simulink library "models2"  (Simulink 6.0)
values from neighbouring files (symbols this model uses):
  width = abs(diff(LTRB(1:2:3)))    [LTRB2Centre.m]
undefined symbols (not defined in the file or in its folder): beta, C, center, coeffs, delG, exponent, i, initialYValues, interact, invcodeData, invDG, knots, m, maxDelay, n, nhi, nk, nlo, numInputSignals, numterms, orderM, paramIndex, poly_order, polycoeff, polyTerms, reorderM, S, s0, s1, sampleTime, target, WendlandNumTerms, Xvalues
libraries: models2 x45, simulink x17
(part 1 of 2)
settings Model: Creator=ralcock  LastModifiedBy=ralcock  ExtModeAutoUpdateStatusClock=off

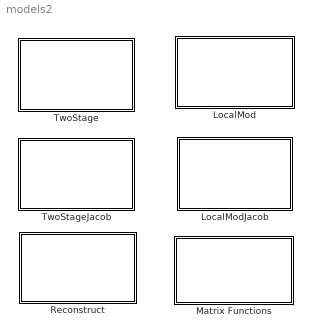
== system models2 ==
  LocalMod : Subsystem
      mask Display: disp('Local Models')
  LocalModJacob : Subsystem
      mask Display: disp('Local Model Jacobians')
  Matrix Functions : Subsystem
      mask Display: disp('Matrix Functions')
  Reconstruct : Subsystem
      mask Display: disp('LocalMod Reconstruct')
  TwoStage : Subsystem
      mask Display: disp('Two Stage models')
  TwoStageJacob : Subsystem
      mask Display: disp('Two Stage Jacobians')

== system models2/LocalMod ==
  expGrowthEval : Subsystem
  gompEval : Subsystem
  localSurfaceCubicEval : Subsystem
  localSurfaceSplineEval : Subsystem  AncestorBlock=models2/TwoStage/xreg3xSplineEval
  localbsplineEval : Subsystem
  logistic4Eval : Subsystem
  logisticEval : Subsystem
  mmfEval : Subsystem
  polynomEval : Subsystem
  polysplineEval : Subsystem
  quadsplineEval : Subsystem
  richardEval : Subsystem
  truncpsEval : Subsystem
  userLocalEval : Subsystem
  weibulEval : Subsystem

== system models2/LocalModJacob ==
  PolynomJacob : Subsystem
  expgrowthJacob : Subsystem
  gompJacob : Subsystem
  localSurfaceCubicJacob : Subsystem  AncestorBlock=models2/TwoStageJacob/xregcubicJacob
  localSurfaceSplineJacob : Subsystem  AncestorBlock=models2/TwoStageJacob/xreg3xsplineJacob
  logistic4Jacob : Subsystem
  logisticJacob : Subsystem
  mmfJacob : Subsystem
  polysplineJacob : Subsystem
  richardJacob : Subsystem
  userLocalJacob : Subsystem
  weibulJacob : Subsystem

== system models2/Matrix Functions ==
  mvMultiplyMatrixSFn : S-Function  FunctionName=mvMultiplyMatrixSFnV1  Parameters=s0,s1
      mask Display: disp('X*Y')
  mvTransposeMatrixSFn : S-Function  FunctionName=mvTransposeMatrixSFnV1  Parameters=s0
      mask Display: disp('X''')

== system models2/Reconstruct ==
  gompRecon : Subsystem
  linearRecon : Subsystem
  localBSplineRecon : Subsystem
  localtruncpsRecon : Subsystem
  log4Recon : Subsystem
  logRecon : Subsystem
  mmfRecon : Subsystem
  richReconDelta : Subsystem
  richReconKappa : Subsystem
  userLocalRecon : Subsystem
  weibRecon : Subsystem

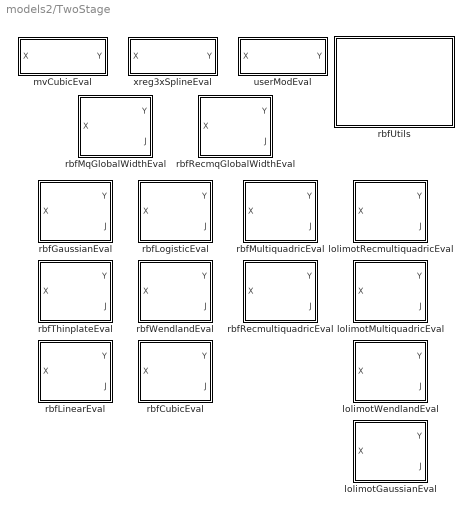
== system models2/TwoStage ==
  lolimotGaussianEval : Subsystem  mask{P=polycoeff, S=width, C=center}
      mask prompts: P "Polynomial coeficients"; S "Widths"; C "Centers"
  lolimotMultiquadricEval : Subsystem  mask{P=polycoeff, S=width, C=center}
      mask prompts: P "Polynomial coeficients"; S "Widths"; C "Centers"
  lolimotRecmultiquadricEval : Subsystem  mask{P=polycoeff, S=width, C=center}
      mask prompts: P "Polynomial coeficients"; S "Widths"; C "Centers"
  lolimotWendlandEval : Subsystem  mask{WendlandNumTerms=WendlandNumTerms, E=exponent, WP=polyTerms, P=polycoeff, S=width, C=center}
      mask prompts: WendlandNumTerms "Number of Polynomial Terms"; E "Exponent"; WP "Polynomial Terms"; P "Polynomial coeficients"; S "Widths"; C "Centers"
  mvCubicEval : Subsystem  AncestorBlock=models2/TwoStage/userModEval
  rbfCubicEval : Subsystem  AncestorBlock=models2/TwoStage/rbfLinearEval  mask{B=beta, S=width, C=center}
      mask prompts: B "Betas"; S "Widths"; C "Centers"
  rbfGaussianEval : Subsystem  mask{B=beta, S=width, C=center}
      mask prompts: B "Betas"; S "Widths"; C "Centers"
  rbfLinearEval : Subsystem  AncestorBlock=models2/TwoStage/rbfThinplateEval  mask{B=beta, S=width, C=center}
      mask prompts: B "Betas"; S "Widths"; C "Centers"
  rbfLogisticEval : Subsystem  mask{B=beta, S=width, C=center}
      mask prompts: B "Betas"; S "Widths"; C "Centers"
  rbfMqGlobalWidthEval : Subsystem  AncestorBlock=models2/TwoStage/rbfMultiquadricEval  mask{B=beta, S=width, C=center}
      mask prompts: B "Betas"; S "Widths"; C "Centers"
  rbfMultiquadricEval : Subsystem  mask{B=beta, S=width, C=center}
      mask prompts: B "Betas"; S "Widths"; C "Centers"
  rbfRecmqGlobalWidthEval : Subsystem  AncestorBlock=models2/TwoStage/rbfRecmultiquadricEval  mask{B=beta, S=width, C=center}
      mask prompts: B "Betas"; S "Widths"; C "Centers"
  rbfRecmultiquadricEval : Subsystem  mask{B=beta, S=width, C=center}
      mask prompts: B "Betas"; S "Widths"; C "Centers"
  rbfThinplateEval : Subsystem  mask{B=beta, S=width, C=center}
      mask prompts: B "Betas"; S "Widths"; C "Centers"
  rbfUtils : Subsystem
      mask Display: disp('RBF Utility blocks')
  rbfWendlandEval : Subsystem  mask{NumTerms=WendlandNumTerms, E=exponent, P=polyTerms, B=beta, S=width, C=center}
      mask prompts: NumTerms "Number of Poylnomial Terms"; E "Exponent"; P "Polynomial Terms"; B "Betas"; S "Widths"; C "Centers"
  userModEval : Subsystem
  xreg3xSplineEval : Subsystem

== system models2/TwoStageJacob ==
  lollimotJacob : Subsystem
  mvcubicJacob : Subsystem
      mask Display: disp('mvCubicJacob')
  rbfJacob : Subsystem
  userModJacob : Subsystem
  xreg3xsplineJacob : Subsystem
      mask Display: disp('xreg3xSplineJacob')
  xregJacob : models2/TwoStageJacob/rbfJacob
  xregcubicJacob : Subsystem  AncestorBlock=models2/TwoStageJacob/mvcubicJacob
      mask Display: disp('mvCubicJacob')
  xreglinear_x2fx : Subsystem
  xregusermodJacob : models2/TwoStageJacob/userModJacob

== system models2/LocalMod/expGrowthEval ==
  P : Inport
  X : Inport  Port=2
  Demux : Demux  Outputs=3
  Gain : Gain  Gain=-1  SaturateOnIntegerOverflow=on
  Math Function : Math  SaturateOnIntegerOverflow=on
  Product : Product  SaturateOnIntegerOverflow=on  InputSameDT=on
  Product1 : Product  SaturateOnIntegerOverflow=on  InputSameDT=on
  Sum : Sum  Inputs=|+-  SaturateOnIntegerOverflow=on  InputSameDT=on
  Sum1 : Sum  Inputs=+-|  SaturateOnIntegerOverflow=on  InputSameDT=on
  Y : Outport
  wires:
  P/1 -> Demux/1
  Demux/2 -> Sum/2  "b"
  Demux/1 -> Sum/1, Sum1/1  "a"
  X/1 -> Product1/2
  Demux/3 -> Gain/1  "k"
  Gain/1 -> Product1/1
  Product1/1 -> Math Function/1
  Math Function/1 -> Product/2
  Sum/1 -> Product/1
  Product/1 -> Sum1/2
  Sum1/1 -> Y/1

== system models2/LocalMod/gompEval ==
  note: a
  note: g
  note: k
  P : Inport
  X : Inport  Port=2
  Demux : Demux  Outputs=3
  Gain : Gain  Gain=-1  SaturateOnIntegerOverflow=on
  Gain1 : Gain  Gain=-1  SaturateOnIntegerOverflow=on
  Math Function : Math  SaturateOnIntegerOverflow=on
  Math Function1 : Math  SaturateOnIntegerOverflow=on
  Product : Product  SaturateOnIntegerOverflow=on  InputSameDT=on
  Product1 : Product  SaturateOnIntegerOverflow=on  InputSameDT=on
  Sum : Sum  Inputs=|-+  SaturateOnIntegerOverflow=on  InputSameDT=on
  Y : Outport
  wires:
  P/1 -> Demux/1
  Demux/2 -> Sum/1
  Demux/3 -> Gain/1
  X/1 -> Sum/2
  Sum/1 -> Product/1
  Gain/1 -> Product/2
  Product/1 -> Math Function/1
  Math Function/1 -> Gain1/1
  Gain1/1 -> Math Function1/1
  Math Function1/1 -> Product1/2
  Demux/1 -> Product1/1
  Product1/1 -> Y/1

== system models2/LocalMod/localSurfaceCubicEval ==
  P : Inport
  X : Inport  Port=2
  Assignment : Assignment  Elements=termsin
  Constant1 : Constant  Value=zeros(1, numterms)
  S-Function : models2/TwoStage/mvCubicEval/S-Function
  Y : Outport
  wires:
  S-Function/1 -> Y/1
  X/1 -> S-Function/2
  P/1 -> Assignment/2
  Assignment/1 -> S-Function/1
  Constant1/1 -> Assignment/1

== system models2/LocalMod/localSurfaceSplineEval ==
  P1 : Inport
  X : Inport  Port=2
  Assignment : Assignment  Elements=termsin
  Constant1 : Constant  Value=zeros(1, numterms)
  S-Function : models2/TwoStage/xreg3xSplineEval/S-Function
  Y : Outport
  wires:
  X/1 -> S-Function/2
  S-Function/1 -> Y/1
  P1/1 -> Assignment/2
  Assignment/1 -> S-Function/1
  Constant1/1 -> Assignment/1

== system models2/LocalMod/localbsplineEval ==
  P : Inport
  X : Inport  Port=2
  S-Function : S-Function  FunctionName=LocalBSplineEvalSFnV1  Parameters="orderm, reorderm,  knots, poly_order, interact, limits"  SFunctionModules=xregsimulinkutils
  Y : Outport
  wires:
  X/1 -> S-Function/2
  S-Function/1 -> Y/1
  P/1 -> S-Function/1

== system models2/LocalMod/logistic4Eval ==
  note: -k * (log(x) - g
  P : Inport
  X : Inport  Port=2
  Constant : Constant
  Demux : Demux
  Gain : Gain  Gain=-1  SaturateOnIntegerOverflow=on
  Math Function : Math  Operator=log  SaturateOnIntegerOverflow=on
  Math Function1 : Math  SaturateOnIntegerOverflow=on
  Product : Product  Inputs=*/  SaturateOnIntegerOverflow=on  InputSameDT=on
  Product1 : Product  SaturateOnIntegerOverflow=on  InputSameDT=on
  Sum : Sum  Inputs=-+|  SaturateOnIntegerOverflow=on  InputSameDT=on
  Sum1 : Sum  Inputs=+-|  SaturateOnIntegerOverflow=on  InputSameDT=on
  Sum2 : Sum  Inputs=|-+  SaturateOnIntegerOverflow=on  InputSameDT=on
  Sum3 : Sum  Inputs=|++  SaturateOnIntegerOverflow=on  InputSameDT=on
  Y : Outport
  wires:
  Demux/2 -> Sum1/1, Sum/2  "b"
  Sum1/1 -> Y/1
  Product/1 -> Sum1/2
  Sum/1 -> Product/1
  Demux/1 -> Sum/1  "a"
  Sum2/1 -> Product1/2
  Math Function/1 -> Sum2/2
  Demux/4 -> Sum2/1  "g"
  Gain/1 -> Product1/1
  Sum3/1 -> Product/2
  Constant/1 -> Sum3/2
  Math Function1/1 -> Sum3/1
  Product1/1 -> Math Function1/1
  Demux/3 -> Gain/1  "k"
  X/1 -> Math Function/1
  P/1 -> Demux/1

== system models2/LocalMod/logisticEval ==
  P : Inport
  X : Inport  Orientation=up  Port=2
  Constant : Constant  Orientation=up
  Demux : Demux  Outputs=3
  Gain : Gain  Gain=-1  SaturateOnIntegerOverflow=on
  Math Function : Math  SaturateOnIntegerOverflow=on
  Product : Product  SaturateOnIntegerOverflow=on  InputSameDT=on
  Product1 : Product  Inputs=*/  SaturateOnIntegerOverflow=on  InputSameDT=on
  Sum : Sum  Inputs=|-+  SaturateOnIntegerOverflow=on  InputSameDT=on
  Sum1 : Sum  Inputs=|++  SaturateOnIntegerOverflow=on  InputSameDT=on
  Y : Outport
  wires:
  P/1 -> Demux/1
  Demux/2 -> Sum/1  "g"
  Demux/3 -> Gain/1  "k"
  X/1 -> Sum/2
  Gain/1 -> Product/2
  Sum/1 -> Product/1
  Product/1 -> Math Function/1
  Math Function/1 -> Sum1/1
  Constant/1 -> Sum1/2
  Sum1/1 -> Product1/2
  Demux/1 -> Product1/1  "a"
  Product1/1 -> Y/1

== system models2/LocalMod/mmfEval ==
  P : Inport
  X : Inport  Orientation=up  Port=2
  Constant : Constant  Orientation=down
  Constant1 : Constant  Orientation=down  Value=NaN
  Constant2 : Constant  Value=0
  Data Type Conversion : DataTypeConversion  OutDataTypeMode=boolean  SaturateOnIntegerOverflow=on  RndMeth=Zero
  Demux : Demux
  Logical Operator : Logic  Operator=OR
  Product : Product  SaturateOnIntegerOverflow=on  InputSameDT=on
  Product1 : Product  Inputs=*/  SaturateOnIntegerOverflow=on  InputSameDT=on
  Relational Operator : RelationalOperator  Operator=<  InputSameDT=on
  SubSystem : Subsystem
  Sum : Sum  Inputs=|+-  SaturateOnIntegerOverflow=on  InputSameDT=on
  Sum2 : Sum  Inputs=+-|  SaturateOnIntegerOverflow=on  InputSameDT=on
  Sum3 : Sum  Inputs=++|  SaturateOnIntegerOverflow=on  InputSameDT=on
  Switch : Switch  Criteria=u2 ~= 0  SaturateOnIntegerOverflow=on  InputSameDT=on
  isComplex : Probe  ProbeWidth=off  ProbeSampleTime=off
  Y : Outport
  wires:
  P/1 -> Demux/1
  Demux/2 -> Sum/2  "b"
  Demux/3 -> Product/1  "k"
  X/1 -> Product/2, Relational Operator/1
  Product/1 -> SubSystem/1(U)
  Sum/1 -> Product1/1
  Product1/1 -> Sum2/2
  Demux/1 -> Sum2/1, Sum/1  "a"
  Demux/4 -> SubSystem/2(V)  "d"
  Switch/1 -> Y/1
  Sum2/1 -> Switch/3, isComplex/1
  Constant1/1 -> Switch/1
  SubSystem/1(U^V) -> Sum3/2
  Constant/1 -> Sum3/1
  Sum3/1 -> Product1/2
  Constant2/1 -> Relational Operator/2
  isComplex/1 -> Data Type Conversion/1
  Logical Operator/1 -> Switch/2
  Relational Operator/1 -> Logical Operator/2
  Data Type Conversion/1 -> Logical Operator/1

== system models2/LocalMod/polynomEval ==
  P : Inport
  X : Inport  Port=2
  polynomEval : S-Function  FunctionName=PolynomEvalSFnV1
  Y : Outport
  wires:
  P/1 -> polynomEval/1
  polynomEval/1 -> Y/1
  X/1 -> polynomEval/2

== system models2/LocalMod/polysplineEval ==
  P : Inport
  X : Inport  Port=2
  datum : Inport  Port=3
  Demux : Demux  Outputs=[1 1 nhi nlo]
  Linear term : Constant  Orientation=down  Value=0
  Mux : Mux  Inputs=3
  Mux1 : Mux  Inputs=3
  Selector : Selector  Elements=[nhi:-1:1]  InputPortWidth=nhi
  Selector1 : Selector  Elements=[nlo:-1:1]  InputPortWidth=nlo
  Sum : Sum  Inputs=-+|  SaturateOnIntegerOverflow=on  InputSameDT=on
  Sum4 : Sum  Inputs=-+|  SaturateOnIntegerOverflow=on  InputSameDT=on
  Switch : Switch  Threshold=eps  InputSameDT=on
  polynomEval1 : S-Function  FunctionName=PolynomEvalSFnV1
  polynomEval2 : S-Function  FunctionName=PolynomEvalSFnV1
  local : Outport
  wires:
  P/1 -> Demux/1
  Demux/3 -> Selector/1  "Phigh"
  Demux/4 -> Selector1/1  "Plow"
  datum/1 -> Sum4/1
  Demux/1 -> Sum4/2  "knot"
  X/1 -> Sum/2
  Sum4/1 -> Sum/1
  Selector/1 -> Mux/1
  Mux/1 -> polynomEval1/1
  Sum/1 -> polynomEval2/2, polynomEval1/2, Switch/2  "X-k"
  Selector1/1 -> Mux1/1
  Mux1/1 -> polynomEval2/1
  Linear term/1 -> Mux/2, Mux1/2
  Demux/2 -> Mux/3, Mux1/3  "P0"
  Switch/1 -> local/1
  polynomEval1/1 -> Switch/1
  polynomEval2/1 -> Switch/3

== system models2/LocalMod/quadsplineEval ==
  note: (X-knot)
  note: (X-knot).^2
  note: quadlow
  note: X
  note: quadhigh
  note: (X-knot).^2
  note: X
  P : Inport
  X : Inport  Port=2
  datum : Inport  Port=3
  Demux : Demux
  Math Function : Math  Operator=square  SaturateOnIntegerOverflow=on
  Math Function1 : Math  Operator=square  SaturateOnIntegerOverflow=on
  Product : Product  SaturateOnIntegerOverflow=on  InputSameDT=on
  Product1 : Product  SaturateOnIntegerOverflow=on  InputSameDT=on
  Sum : Sum  Inputs=|+-  SaturateOnIntegerOverflow=on  InputSameDT=on
  Sum1 : Sum  Inputs=|++  SaturateOnIntegerOverflow=on  InputSameDT=on
  Sum2 : Sum  Inputs=-+|  SaturateOnIntegerOverflow=on  InputSameDT=on
  Sum3 : Sum  Inputs=++|  SaturateOnIntegerOverflow=on  InputSameDT=on
  Sum4 : Sum  Inputs=-+|  SaturateOnIntegerOverflow=on  InputSameDT=on
  Switch : Switch  Threshold=eps  InputSameDT=on
  local : Outport
  wires:
  Switch/1 -> local/1
  Sum/1 -> Switch/2, Math Function/1
  Product1/1 -> Sum3/2
  Demux/4 -> Product1/1  "Plow"
  Math Function1/1 -> Product1/2
  Sum2/1 -> Math Function1/1
  X/1 -> Sum2/2, Sum/1
  Product/1 -> Sum1/1
  Demux/3 -> Product/2  "Phigh"
  P/1 -> Demux/1
  Math Function/1 -> Product/1
  Demux/2 -> Sum3/1, Sum1/2  "P0"
  Sum3/1 -> Switch/3
  Sum1/1 -> Switch/1
  Demux/1 -> Sum4/2  "knot"
  datum/1 -> Sum4/1
  Sum4/1 -> Sum/2, Sum2/1

== system models2/LocalMod/richardEval ==
  note: The Tolerance block triggers when
      | d is within 3e-6 of 1. See notes from
      |  TM for a definition of the limit at d =1
  P : Inport
  X : Inport  Port=2
  Complex to Real-Imag : ComplexToRealImag  Output=Real
  Complex to Real-Imag1 : ComplexToRealImag  Output=Imag
  Constant1 : Constant  Orientation=down  Value=NaN + i
  Data Type Conversion : DataTypeConversion  OutDataTypeMode=boolean  SaturateOnIntegerOverflow=on  RndMeth=Zero
  Demux1 : Demux
  Logical Operator : Logic  Operator=NOT
  Richards : Subsystem  TreatAsAtomicUnit=on
  Richards  at d == 1 : Subsystem  TreatAsAtomicUnit=on
  SubSystem : models2/LocalModJacob/richardJacob/SubSystem  V=1  T=3e-6
  Switch : Switch  Threshold=0.5  InputSameDT=on
  Switch1 : Switch  Criteria=u2 ~= 0  SaturateOnIntegerOverflow=on  InputSameDT=on
  Terminator1 : Terminator
  Terminator2 : Terminator
  Terminator3 : Terminator
  Y : Outport
  wires:
  Demux1/4 -> SubSystem/1  "d"
  P/1 -> Richards/1(P), Richards  at d == 1/1(P), Demux1/1
  X/1 -> Richards/2(X), Richards  at d == 1/2(X)
  Richards  at d == 1/1(Y) -> Switch/3
  Richards/1(Y) -> Switch/1
  Demux1/1 -> Terminator2/1  "a"
  Demux1/2 -> Terminator1/1  "g"
  Demux1/3 -> Terminator3/1  "k"
  SubSystem/1 -> Logical Operator/1, Richards  at d == 1/Enable
  Logical Operator/1 -> Switch/2, Richards/Enable
  Switch1/1 -> Complex to Real-Imag/1
  Constant1/1 -> Switch1/1
  Complex to Real-Imag1/1 -> Data Type Conversion/1
  Switch/1 -> Switch1/3, Complex to Real-Imag1/1
  Data Type Conversion/1 -> Switch1/2
  Complex to Real-Imag/1 -> Y/1

== system models2/LocalMod/truncpsEval ==
  P : Inport
  X : Inport  Port=2
  Constant1 : Constant  Value=m
  Constant2 : Constant  Value=0
  Demux : Demux  Outputs=[nk n-2*nk nk]
  Dot Product : simulink/Math Operations/Dot Product  OutDataType=sfix(16)  OutScaling=2^-10  DoSatur=off
  Math Function : Math  Operator=pow  SaturateOnIntegerOverflow=on
  Sum : Sum  Inputs=|+-  SaturateOnIntegerOverflow=on  InputSameDT=on
  Sum2 : Sum  Inputs=++|  SaturateOnIntegerOverflow=on  InputSameDT=on
  Switch : Switch  InputSameDT=on
  polyval : S-Function  FunctionName=PolynomEvalSFnV1
  y : Outport
  wires:
  Demux/2 -> polyval/1  "b_poly"
  Sum2/1 -> y/1
  polyval/1 -> Sum2/1
  Constant1/1 -> Math Function/2
  Switch/1 -> Math Function/1
  Dot Product/1 -> Sum2/2
  Math Function/1 -> Dot Product/1
  Demux/3 -> Dot Product/2  "bspline"
  Constant2/1 -> Switch/3
  X/1 -> Sum/1, polyval/2
  Sum/1 -> Switch/2, Switch/1
  P/1 -> Demux/1
  Demux/1 -> Sum/2  "knots"

== system models2/LocalMod/userLocalEval ==
  P : Inport
  X : Inport  Port=2
  Y : Outport

== system models2/LocalMod/weibulEval ==
  P : Inport
  X : Inport  Orientation=up  Port=2
  Constant1 : Constant  Orientation=down  Value=NaN
  Constant2 : Constant  Value=0
  Data Type Conversion : DataTypeConversion  OutDataTypeMode=boolean  SaturateOnIntegerOverflow=on  RndMeth=Zero
  Demux : Demux
  Logical Operator : Logic  Operator=OR
  Product : Product  SaturateOnIntegerOverflow=on  InputSameDT=on
  Product1 : Product  SaturateOnIntegerOverflow=on  InputSameDT=on
  Relational Operator : RelationalOperator  Operator=<  InputSameDT=on
  SubSystem : Subsystem
  Sum : Sum  Inputs=+-|  SaturateOnIntegerOverflow=on  InputSameDT=on
  Sum1 : Sum  Inputs=+-|  SaturateOnIntegerOverflow=on  InputSameDT=on
  Switch : Switch  Criteria=u2 ~= 0  SaturateOnIntegerOverflow=on  InputSameDT=on
  isComplex : Probe  ProbeWidth=off  ProbeSampleTime=off
  Y : Outport
  wires:
  Product1/1 -> Sum1/2
  Sum/1 -> Product1/1
  SubSystem/1(e^-(U^V)) -> Product1/2  "-(k*x) ^ d"
  Product/1 -> SubSystem/1(U)
  Demux/1 -> Sum1/1, Sum/1  "a"
  Demux/2 -> Sum/2  "b"
  Demux/4 -> SubSystem/2(V)  "d"
  X/1 -> Product/2, Relational Operator/1
  Demux/3 -> Product/1  "k"
  P/1 -> Demux/1
  Constant1/1 -> Switch/1
  isComplex/1 -> Data Type Conversion/1
  Logical Operator/1 -> Switch/2
  Constant2/1 -> Relational Operator/2
  Sum1/1 -> Switch/3, isComplex/1
  Switch/1 -> Y/1
  Relational Operator/1 -> Logical Operator/2
  Data Type Conversion/1 -> Logical Operator/1

== system models2/LocalModJacob/PolynomJacob ==
  P : Inport
  X : Inport  Port=2
  PolynomJacob : S-Function  FunctionName=PolynomJacobSFnV1
  J : Outport
  wires:
  PolynomJacob/1 -> J/1
  X/1 -> PolynomJacob/2
  P/1 -> PolynomJacob/1

== system models2/LocalModJacob/expgrowthJacob ==
  P : Inport
  X : Inport  Port=2
  Constant : Constant
  Demux : Demux  Outputs=3
  Gain : Gain  Gain=-1  SaturateOnIntegerOverflow=on
  Gain3 : Gain  Gain=-1  SaturateOnIntegerOverflow=on
  Math Function : Math  SaturateOnIntegerOverflow=on
  Mux : Mux  Inputs=3
  Product1 : Product  SaturateOnIntegerOverflow=on  InputSameDT=on
  Product2 : Product  Inputs=3  SaturateOnIntegerOverflow=on  InputSameDT=on
  Sum : Sum  Inputs=|+-  SaturateOnIntegerOverflow=on  InputSameDT=on
  Sum1 : Sum  Inputs=|+-  SaturateOnIntegerOverflow=on  InputSameDT=on
  J : Outport
  wires:
  Demux/3 -> Gain/1  "k"
  Demux/1 -> Sum/1  "a"
  Demux/2 -> Sum/2  "b"
  Sum1/1 -> Mux/1  "Ja"
  Sum/1 -> Product2/3
  X/1 -> Product1/2, Product2/2
  Product2/1 -> Mux/3  "Jk"
  Gain/1 -> Product1/1
  Product1/1 -> Math Function/1
  Math Function/1 -> Sum1/2, Mux/2, Product2/1  "Jb"
  Gain3/1 -> J/1
  Mux/1 -> Gain3/1
  P/1 -> Demux/1
  Constant/1 -> Sum1/1

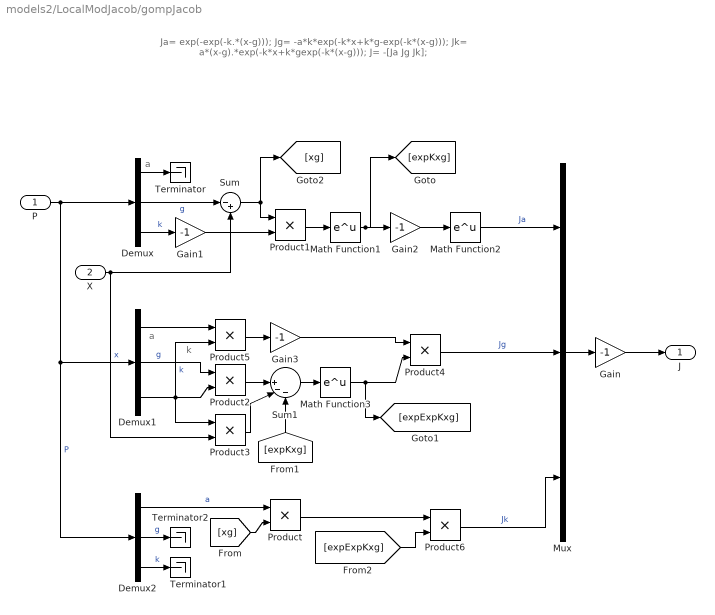
== system models2/LocalModJacob/gompJacob ==
  note: Ja= exp(-exp(-k.*(x-g)));
      | Jg= -a*k*exp(-k*x+k*g-exp(-k*(x-g)));
      | Jk= a*(x-g).*exp(-k*x+k*gexp(-k*(x-g)));
      |
      | J= -[Ja Jg Jk];
  note: a
  note: a
  note: k
  P : Inport
  X : Inport  Port=2
  Demux : Demux  Outputs=3
  Demux1 : Demux  Outputs=3
  Demux2 : Demux  Outputs=3
  Gain{,1..3} (4 alike) : Gain  Gain=-1  SaturateOnIntegerOverflow=on
  Math Function1 : Math  SaturateOnIntegerOverflow=on
  Math Function2 : Math  SaturateOnIntegerOverflow=on
  Math Function3 : Math  SaturateOnIntegerOverflow=on
  Mux : Mux  Inputs=3
  Product{,1..6} (7 alike) : Product  SaturateOnIntegerOverflow=on  InputSameDT=on
  Sum : Sum  Inputs=|-+  SaturateOnIntegerOverflow=on  InputSameDT=on
  Sum1 : Sum  Inputs=||+--  SaturateOnIntegerOverflow=on  InputSameDT=on
  Terminator : Terminator
  Terminator1 : Terminator
  Terminator2 : Terminator
  J : Outport
  wires:
  Gain/1 -> J/1
  Demux/1 -> Terminator/1
  Demux/2 -> Sum/1  "g"
  Product1/1 -> Math Function1/1
  Demux/3 -> Gain1/1  "k"
  Gain1/1 -> Product1/2
  Gain2/1 -> Math Function2/1
  Math Function1/1 -> Gain2/1, [expKxg]
  P/1 -> Demux/1, Demux1/1, Demux2/1  "P"
  X/1 -> Sum/2, Product3/2  "x"
  Sum/1 -> Product1/1, [xg]
  Demux2/3 -> Terminator1/1  "k"
  Demux2/2 -> Terminator2/1  "g"
  Demux2/1 -> Product/1  "a"
  [xg] -> Product/2
  Product/1 -> Product6/1
  [expExpKxg] -> Product6/2
  Product6/1 -> Mux/3  "Jk"
  Math Function2/1 -> Mux/1  "Ja"
  Mux/1 -> Gain/1
  Demux1/2 -> Product2/1  "g"
  Product2/1 -> Sum1/1
  [expKxg] -> Sum1/3
  Demux1/3 -> Product3/1, Product2/2, Product5/2  "k"
  Product3/1 -> Sum1/2
  Sum1/1 -> Math Function3/1
  Math Function3/1 -> [expExpKxg], Product4/2
  Demux1/1 -> Product5/1
  Product5/1 -> Gain3/1
  Gain3/1 -> Product4/1
  Product4/1 -> Mux/2  "Jg"

== system models2/LocalModJacob/localSurfaceCubicJacob ==
  P1 : Inport
  X : Inport  Port=2
  Assignment : Assignment  Elements=termsin
  Constant1 : Constant  Value=zeros(1, numterms)
  S-Function : models2/TwoStageJacob/xregcubicJacob/S-Function
  Selector1 : Selector  Elements=termsout  InputPortWidth=numterms
  J : Outport
  wires:
  S-Function/1 -> Selector1/1
  X/1 -> S-Function/2
  Selector1/1 -> J/1
  P1/1 -> Assignment/2
  Assignment/1 -> S-Function/1
  Constant1/1 -> Assignment/1

== system models2/LocalModJacob/localSurfaceSplineJacob ==
  P : Inport
  X : Inport  Port=2
  Assignment : Assignment  Elements=termsin
  Constant1 : Constant  Value=zeros(1, numterms)
  S-Function : models2/TwoStageJacob/xreg3xsplineJacob/S-Function
  Selector1 : Selector  Elements=termsout  InputPortWidth=numterms
  J : Outport
  wires:
  S-Function/1 -> Selector1/1
  X/1 -> S-Function/2
  Selector1/1 -> J/1
  P/1 -> Assignment/2
  Assignment/1 -> S-Function/1
  Constant1/1 -> Assignment/1

== system models2/LocalModJacob/logistic4Jacob ==
  P : Inport
  X : Inport  Port=2
  Constant : Constant  Orientation=down
  Demux : Demux
  Demux1 : Demux  Outputs=3
  Gain : Gain  Gain=-1  SaturateOnIntegerOverflow=on
  Gain2 : Gain  Gain=-1  SaturateOnIntegerOverflow=on
  Math Function : Math  Operator=log  SaturateOnIntegerOverflow=on
  Mux : Mux  Inputs=3
  Mux1 : Mux
  Sum : Sum  Inputs=-+|  SaturateOnIntegerOverflow=on  InputSameDT=on
  Sum1 : Sum  Inputs=-+|  SaturateOnIntegerOverflow=on  InputSameDT=on
  logisticJacob : Subsystem
  J : Outport
  wires:
  P/1 -> Demux/1
  Demux/1 -> Sum/1  "a"
  Demux/2 -> Sum/2  "b"
  Sum/1 -> Mux/1  "a'"
  Mux/1 -> logisticJacob/1(P)
  Demux/3 -> Mux/3  "k"
  Demux/4 -> Mux/2  "g"
  X/1 -> Math Function/1
  Math Function/1 -> logisticJacob/2(X)
  Demux1/1 -> Sum1/2, Gain/1  "Ja"
  Constant/1 -> Sum1/1
  Sum1/1 -> Mux1/2  "Jb"
  Mux1/1 -> J/1
  Demux1/2 -> Mux1/4  "Jg"
  Demux1/3 -> Mux1/3  "Jk"
  Gain/1 -> Mux1/1  "Ja"
  logisticJacob/1(J) -> Gain2/1
  Gain2/1 -> Demux1/1  "Ja"

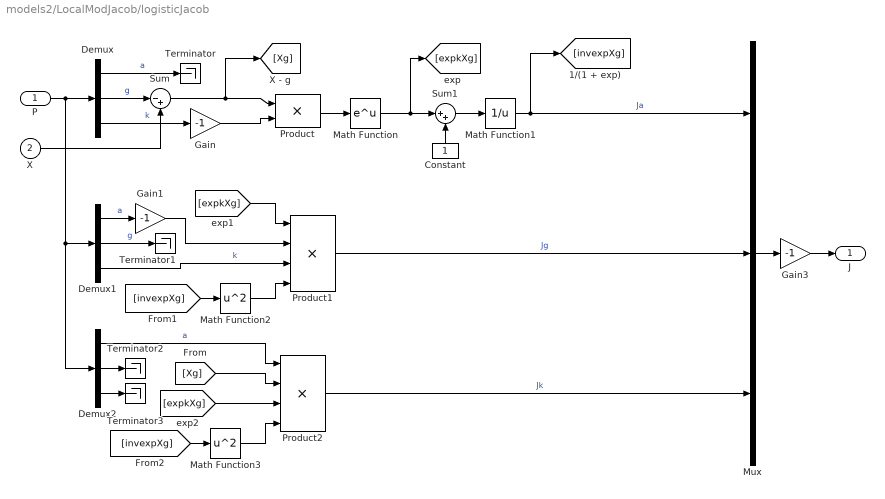
== system models2/LocalModJacob/logisticJacob ==
  P : Inport
  X : Inport  Port=2
  Constant : Constant  Orientation=up
  Demux : Demux  Outputs=3
  Demux1 : Demux  Outputs=3
  Demux2 : Demux  Outputs=3
  Gain : Gain  Gain=-1  SaturateOnIntegerOverflow=on
  Gain1 : Gain  Gain=-1  SaturateOnIntegerOverflow=on
  Gain3 : Gain  Gain=-1  SaturateOnIntegerOverflow=on
  Math Function : Math  SaturateOnIntegerOverflow=on
  Math Function1 : Math  Operator=reciprocal  OutputSignalType=real  SaturateOnIntegerOverflow=on
  Math Function2 : Math  Operator=square  SaturateOnIntegerOverflow=on
  Math Function3 : Math  Operator=square  SaturateOnIntegerOverflow=on
  Mux : Mux  Inputs=3
  Product : Product  SaturateOnIntegerOverflow=on  InputSameDT=on
  Product1 : Product  Inputs=4  SaturateOnIntegerOverflow=on  InputSameDT=on
  Product2 : Product  Inputs=4  SaturateOnIntegerOverflow=on  InputSameDT=on
  Sum : Sum  Inputs=|-+  SaturateOnIntegerOverflow=on  InputSameDT=on
  Sum1 : Sum  Inputs=|++  SaturateOnIntegerOverflow=on  InputSameDT=on
  Terminator{,1..3} (4 alike) : Terminator
  J : Outport
  wires:
  P/1 -> Demux/1, Demux1/1, Demux2/1
  Demux/1 -> Terminator/1  "a"
  Demux/2 -> Sum/1  "g"
  X/1 -> Sum/2
  Sum/1 -> Product/1, [Xg]
  Demux/3 -> Gain/1  "k"
  Gain/1 -> Product/2
  Product/1 -> Math Function/1
  Math Function/1 -> [expkXg], Sum1/1
  Constant/1 -> Sum1/2
  Sum1/1 -> Math Function1/1
  Demux1/1 -> Gain1/1  "a"
  Gain1/1 -> Product1/2
  Demux1/2 -> Terminator1/1  "g"
  [expkXg] -> Product1/1
  [invexpXg] -> Math Function2/1
  Math Function1/1 -> [invexpXg], Mux/1  "Ja"
  Math Function2/1 -> Product1/4
  Product1/1 -> Mux/2  "Jg"
  Mux/1 -> Gain3/1
  Gain3/1 -> J/1
  Demux1/3 -> Product1/3  "k"
  Demux2/2 -> Terminator2/1
  Demux2/3 -> Terminator3/1
  Demux2/1 -> Product2/1  "a"
  [invexpXg] -> Math Function3/1
  [Xg] -> Product2/2
  Product2/1 -> Mux/3  "Jk"
  [expkXg] -> Product2/3
  Math Function3/1 -> Product2/4

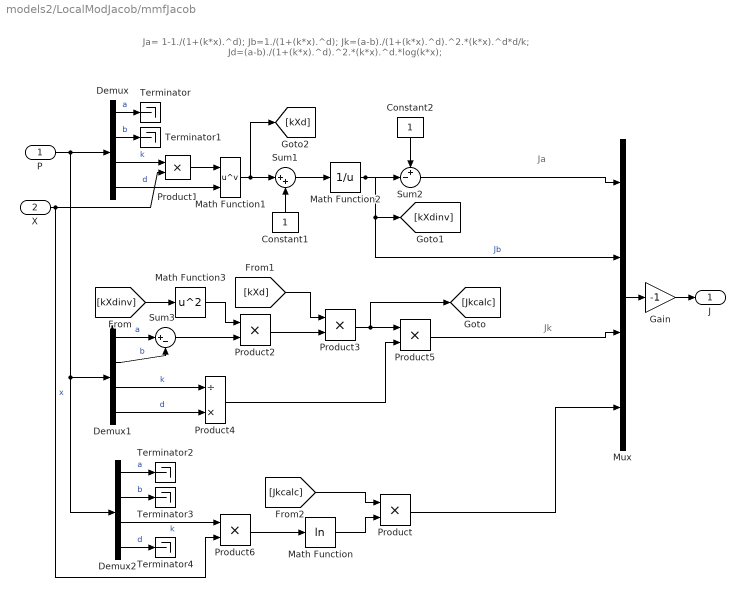
== system models2/LocalModJacob/mmfJacob ==
  note: Jk
  note: Ja
  note: Ja= 1-1./(1+(k*x).^d);
      | Jb=1./(1+(k*x).^d);
      | Jk=(a-b)./(1+(k*x).^d).^2.*(k*x).^d*d/k;
      | Jd=(a-b)./(1+(k*x).^d).^2.*(k*x).^d.*log(k*x);
  P : Inport
  X : Inport  Port=2
  Constant1 : Constant  Orientation=up
  Constant2 : Constant  Orientation=down
  Demux : Demux
  Demux1 : Demux
  Demux2 : Demux
  Gain : Gain  Gain=-1  SaturateOnIntegerOverflow=on
  Math Function : Math  Operator=log  SaturateOnIntegerOverflow=on
  Math Function1 : Math  Operator=pow  SaturateOnIntegerOverflow=on
  Math Function2 : Math  Operator=reciprocal  SaturateOnIntegerOverflow=on
  Math Function3 : Math  Operator=square  SaturateOnIntegerOverflow=on
  Mux : Mux
  Product{,1..3,5..6} (6 alike) : Product  SaturateOnIntegerOverflow=on  InputSameDT=on
  Product4 : Product  Inputs=/*  SaturateOnIntegerOverflow=on  InputSameDT=on
  Sum1 : Sum  Inputs=|++  SaturateOnIntegerOverflow=on  InputSameDT=on
  Sum2 : Sum  Inputs=+-|  SaturateOnIntegerOverflow=on  InputSameDT=on
  Sum3 : Sum  Inputs=|+-  SaturateOnIntegerOverflow=on  InputSameDT=on
  Terminator{,1..4} (5 alike) : Terminator
  J : Outport
  wires:
  Gain/1 -> J/1
  Mux/1 -> Gain/1
  Product/1 -> Mux/4
  Product5/1 -> Mux/3
  [Jkcalc] -> Product/1
  Math Function/1 -> Product/2
  Product6/1 -> Math Function/1
  Demux2/3 -> Product6/1  "k"
  Demux2/4 -> Terminator4/1  "d"
  Demux2/2 -> Terminator3/1  "b"
  Demux2/1 -> Terminator2/1  "a"
  X/1 -> Product6/2, Product1/2  "x"
  Product3/1 -> [Jkcalc], Product5/1
  Product4/1 -> Product5/2
  Demux1/4 -> Product4/2  "d"
  Demux1/3 -> Product4/1  "k"
  [kXd] -> Product3/1
  Product2/1 -> Product3/2
  Math Function3/1 -> Product2/1
  [kXdinv] -> Math Function3/1
  Sum3/1 -> Product2/2
  Demux1/1 -> Sum3/1  "a"
  Demux1/2 -> Sum3/2  "b"
  Math Function1/1 -> [kXd], Sum1/1
  P/1 -> Demux2/1, Demux1/1, Demux/1
  Constant2/1 -> Sum2/1
  Math Function2/1 -> Mux/2, [kXdinv], Sum2/2  "Jb"
  Sum2/1 -> Mux/1
  Sum1/1 -> Math Function2/1
  Constant1/1 -> Sum1/2
  Product1/1 -> Math Function1/1
  Demux/3 -> Product1/1  "k"
  Demux/4 -> Math Function1/2  "d"
  Demux/2 -> Terminator1/1  "b"
  Demux/1 -> Terminator/1  "a"

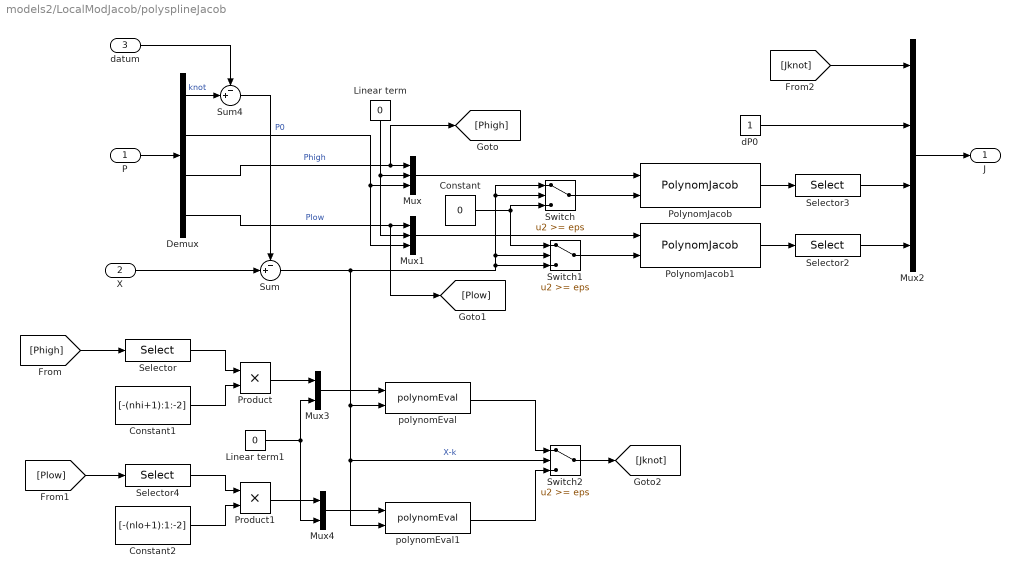
== system models2/LocalModJacob/polysplineJacob ==
  P : Inport
  X : Inport  Port=2
  datum : Inport  Port=3
  Constant : Constant  Value=0
  Constant1 : Constant  Value=[-(nhi+1):1:-2]
  Constant2 : Constant  Value=[-(nlo+1):1:-2]
  Demux : Demux  Outputs=[1 1 nhi nlo]
  Linear term : Constant  Orientation=down  Value=0
  Linear term1 : Constant  Value=0
  Mux : Mux  Inputs=3
  Mux1 : Mux  Inputs=3
  Mux2 : Mux  Inputs=[1 1 nhi nlo]
  Mux3 : Mux  Inputs=2
  Mux4 : Mux  Inputs=2
  PolynomJacob : models2/LocalModJacob/PolynomJacob
  PolynomJacob1 : models2/LocalModJacob/PolynomJacob
  Product : Product  SaturateOnIntegerOverflow=on  InputSameDT=on
  Product1 : Product  SaturateOnIntegerOverflow=on  InputSameDT=on
  Selector : Selector  Elements=[nhi:-1:1]  InputPortWidth=nhi
  Selector2 : Selector  Elements=[nlo:-1:1]  InputPortWidth=nlo+2
  Selector3 : Selector  Elements=[nhi:-1:1]  InputPortWidth=nhi+2
  Selector4 : Selector  Elements=[nlo:-1:1]  InputPortWidth=nlo
  Sum : Sum  Inputs=-+|  SaturateOnIntegerOverflow=on  InputSameDT=on
  Sum4 : Sum  Inputs=-+|  SaturateOnIntegerOverflow=on  InputSameDT=on
  Switch : Switch  Threshold=eps  InputSameDT=on
  Switch1 : Switch  Threshold=eps  InputSameDT=on
  Switch2 : Switch  Threshold=eps  InputSameDT=on
  dP0 : Constant
  polynomEval : models2/LocalMod/polynomEval
  polynomEval1 : models2/LocalMod/polynomEval
  J : Outport
  wires:
  Demux/4 -> [Plow], Mux1/1  "Plow"
  Demux/3 -> [Phigh], Mux/1  "Phigh"
  Selector3/1 -> Mux2/3
  PolynomJacob/1 -> Selector3/1
  Selector2/1 -> Mux2/4
  PolynomJacob1/1 -> Selector2/1
  Mux2/1 -> J/1
  [Jknot] -> Mux2/1
  Switch2/1 -> [Jknot]
  polynomEval1/1 -> Switch2/3
  polynomEval/1 -> Switch2/1
  Sum/1 -> Switch2/2, polynomEval1/2, polynomEval/2, Switch1/3, Switch1/2, Switch/1, Switch/2  "X-k"
  Mux4/1 -> polynomEval1/1
  Mux3/1 -> polynomEval/1
  Linear term1/1 -> Mux4/2, Mux3/2
  Product1/1 -> Mux4/1
  Product/1 -> Mux3/1
  Constant1/1 -> Product/2
  dP0/1 -> Mux2/2
  Sum4/1 -> Sum/1
  X/1 -> Sum/2
  Mux/1 -> PolynomJacob/1
  Switch/1 -> PolynomJacob/2
  Mux1/1 -> PolynomJacob1/1
  Switch1/1 -> PolynomJacob1/2
  Demux/1 -> Sum4/2  "knot"
  datum/1 -> Sum4/1
  Demux/2 -> Mux/3, Mux1/3  "P0"
  P/1 -> Demux/1
  Constant/1 -> Switch1/1, Switch/3
  Linear term/1 -> Mux/2, Mux1/2
  [Phigh] -> Selector/1
  Selector/1 -> Product/1
  [Plow] -> Selector4/1
  Selector4/1 -> Product1/1
  Constant2/1 -> Product1/2

== system models2/LocalModJacob/richardJacob ==
  note: The Tolerance block triggers when
      | d is within 3e-6 of 1. See notes from
      |  TM for a definition of the limit at d =1
  P : Inport
  X : Inport  Port=2
  Demux1 : Demux
  Gain1 : Gain  Gain=-1  SaturateOnIntegerOverflow=on
  Logical Operator : Logic  Operator=NOT
  Richards Jacobian : Subsystem  TreatAsAtomicUnit=on
  Richards Jacobian at d = 1 : Subsystem  TreatAsAtomicUnit=on
  SubSystem : Subsystem  mask{V=1, T=3e-6}
      mask prompts: V "Value to compare"; T "Tolerance"
      mask Display: disp('Tol')
  Switch : Switch  Threshold=0.5  InputSameDT=on
  Terminator1 : Terminator
  Terminator2 : Terminator
  Terminator3 : Terminator
  J : Outport
  wires:
  Demux1/4 -> SubSystem/1(I)  "d"
  P/1 -> Richards Jacobian/1(P), Richards Jacobian at d = 1/1(P), Demux1/1
  X/1 -> Richards Jacobian/2(X), Richards Jacobian at d = 1/2(X)
  Gain1/1 -> J/1
  Switch/1 -> Gain1/1
  Richards Jacobian at d = 1/1(J) -> Switch/3
  Richards Jacobian/1(J) -> Switch/1
  Demux1/1 -> Terminator2/1  "a"
  Demux1/2 -> Terminator1/1  "g"
  Demux1/3 -> Terminator3/1  "k"
  SubSystem/1(Out) -> Logical Operator/1, Richards Jacobian at d = 1/Enable
  Logical Operator/1 -> Switch/2, Richards Jacobian/Enable

== system models2/LocalModJacob/userLocalJacob ==
  P : Inport
  X : Inport  Port=2
  J : Outport

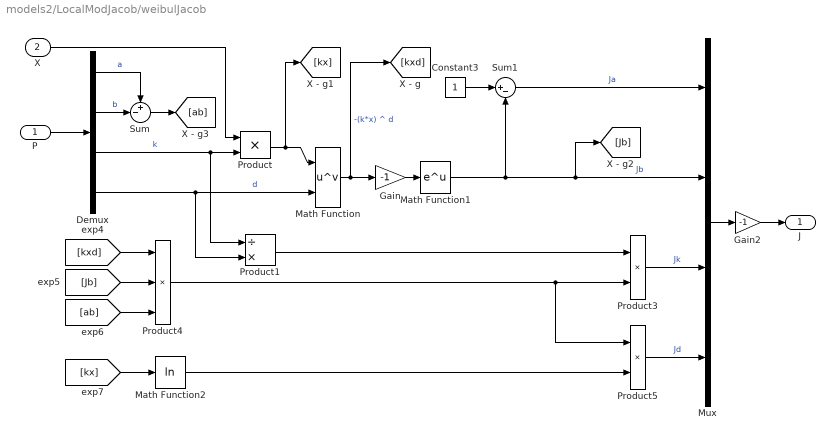
== system models2/LocalModJacob/weibulJacob ==
  P : Inport
  X : Inport  Port=2
  Constant3 : Constant
  Demux : Demux
  Gain : Gain  Gain=-1  SaturateOnIntegerOverflow=on
  Gain2 : Gain  Gain=-1  SaturateOnIntegerOverflow=on
  Math Function : Math  Operator=pow  SaturateOnIntegerOverflow=on
  Math Function1 : Math  SaturateOnIntegerOverflow=on
  Math Function2 : Math  Operator=log  SaturateOnIntegerOverflow=on
  Mux : Mux
  Product : Product  SaturateOnIntegerOverflow=on  InputSameDT=on
  Product1 : Product  Inputs=/*  SaturateOnIntegerOverflow=on  InputSameDT=on
  Product3 : Product  SaturateOnIntegerOverflow=on  InputSameDT=on
  Product4 : Product  Inputs=3  SaturateOnIntegerOverflow=on  InputSameDT=on
  Product5 : Product  SaturateOnIntegerOverflow=on  InputSameDT=on
  Sum : Sum  Inputs=+-|  SaturateOnIntegerOverflow=on  InputSameDT=on
  Sum1 : Sum  Inputs=|+-  SaturateOnIntegerOverflow=on  InputSameDT=on
  J : Outport
  wires:
  Demux/2 -> Sum/2  "b"
  P/1 -> Demux/1
  Demux/1 -> Sum/1  "a"
  Sum/1 -> [ab]
  Gain/1 -> Math Function1/1
  Math Function/1 -> Gain/1, [kxd]  "-(k*x) ^ d"
  X/1 -> Product/1
  Product/1 -> Math Function/1, [kx]
  Constant3/1 -> Sum1/1
  Sum1/1 -> Mux/1  "Ja"
  Math Function1/1 -> Sum1/2, Mux/2, [Jb]  "Jb"
  Product3/1 -> Mux/3  "Jk"
  Demux/3 -> Product/2, Product1/1  "k"
  Demux/4 -> Math Function/2, Product1/2  "d"
  [kxd] -> Product4/1
  [Jb] -> Product4/2
  [ab] -> Product4/3
  Product1/1 -> Product3/1
  Product5/1 -> Mux/4  "Jd"
  [kx] -> Math Function2/1
  Math Function2/1 -> Product5/2
  Product4/1 -> Product3/2, Product5/1
  Mux/1 -> Gain2/1
  Gain2/1 -> J/1

== system models2/Reconstruct/gompRecon ==
  Param : Inport
  Ground : Ground
  Linear  Reconstruct : Gain  Gain=invDG  Multiplication=Matrix(K*u)  SaturateOnIntegerOverflow=on
  Linear Terms : Selector  Elements=LinTerms  InputPortWidth=NTerms
  Mux : Mux  Inputs=2
  Mux1 : Mux  Inputs=2
  Nonlinear Terms : Selector  Elements=NLTerm  InputPortWidth=NTerms
  Nonlinear reconstruct : Subsystem
  Pn : Selector  Orientation=down  Elements=KnownParam  InputPortWidth=NTerms
  Recombine : Selector  Elements=recombine  InputPortWidth=NTerms
  Param Rec : Outport
  h : Outport  Port=2
  wires:
  Nonlinear reconstruct/1(k) -> Mux/2
  Param/1 -> Linear  Reconstruct/1, Nonlinear Terms/1
  Linear  Reconstruct/1 -> Pn/1, Linear Terms/1
  Linear Terms/1 -> Mux/1
  Nonlinear Terms/1 -> Mux1/2
  Pn/1 -> Mux1/1  "P"
  Mux1/1 -> Nonlinear reconstruct/1(P)
  Mux/1 -> Recombine/1
  Recombine/1 -> Param Rec/1
  Ground/1 -> h/1

== system models2/Reconstruct/linearRecon ==
  Param : Inport
  Constant : Constant  Value=invDG(:)
  Linear Reconstruct : Gain  Gain=invDG  Multiplication=Matrix(K*u)  SaturateOnIntegerOverflow=on
  Param Rec : Outport
  h : Outport  Port=2
  wires:
  Linear Reconstruct/1 -> Param Rec/1
  Param/1 -> Linear Reconstruct/1
  Constant/1 -> h/1

== system models2/Reconstruct/localBSplineRecon ==
  Param : Inport
  Code : Subsystem
  Ground : Ground
  Mux : Mux  Inputs=2
  PhiCalc : Subsystem
  Product : Product  Inputs=/*  Multiplication=Matrix(*)  SaturateOnIntegerOverflow=on  InputSameDT=on
  S-Function : S-Function  FunctionName=qsortSFnV1
  Saturation : Saturate  UpperLimit=target(2)- sqrt(eps)*max(abs(target))  LowerLimit=target(1)+ sqrt(eps)*max(abs(target))
  Select knots : Selector  Elements=knots
  Select params : Selector  Elements=params
  Xvalues : Constant  Value=Xvalues
  Param Rec : Outport
  h : Outport  Port=2
  wires:
  Param/1 -> Select knots/1, Select params/1
  Select knots/1 -> Code/1(K)
  Code/1(Coded K) -> S-Function/1
  Xvalues/1 -> PhiCalc/2(X)
  PhiCalc/1(delG) -> Product/1
  Select params/1 -> Product/2
  Product/1 -> Mux/2
  Mux/1 -> Param Rec/1
  Ground/1 -> h/1
  Saturation/1 -> PhiCalc/1(knots), Mux/1
  S-Function/1 -> Saturation/1

== system models2/Reconstruct/localtruncpsRecon ==
  Param : Inport
  Code : Subsystem
  Ground : Ground
  Mux : Mux  Inputs=2
  Product : Product  Inputs=/*  Multiplication=Matrix(*)  SaturateOnIntegerOverflow=on  InputSameDT=on
  S-Function : S-Function  FunctionName=qsortSFnV1
  Select knots : Selector  Elements=knots
  Select params : Selector  Elements=params
  fill dG : Subsystem
  Param Rec : Outport
  h : Outport  Port=2
  wires:
  Ground/1 -> h/1
  Mux/1 -> Param Rec/1
  Product/1 -> Mux/2
  Select params/1 -> Product/2
  fill dG/1(delG) -> Product/1
  Code/1(Coded K) -> S-Function/1
  Select knots/1 -> Code/1(K)
  Param/1 -> Select params/1, Select knots/1
  S-Function/1 -> fill dG/1(knots), Mux/1

== system models2/Reconstruct/log4Recon ==
  Param : Inport
  Ground : Ground
  Linear Reconstruct : Gain  Gain=invDG  Multiplication=Matrix(K*u)  SaturateOnIntegerOverflow=on
  Linear Terms : Selector  Elements=Log4LinTerms  InputPortWidth=NTerms
  Mux : Mux  Inputs=2
  Mux1 : Mux  Inputs=2
  Nonlinear (Kappa)  reconstruct : Subsystem
  Nonlinear Terms : Selector  Elements=NLTerm  InputPortWidth=NTerms
  P3 : Selector  Orientation=down  Elements=3  InputPortWidth=NTerms
  recombine : Selector  Elements=recombine  InputPortWidth=NTerms
  Param Rec : Outport
  h : Outport  Port=2
  wires:
  Nonlinear (Kappa)  reconstruct/1(K) -> Mux/2
  Param/1 -> Linear Reconstruct/1, Nonlinear Terms/1
  Mux1/1 -> Nonlinear (Kappa)  reconstruct/1(P)
  Nonlinear Terms/1 -> Mux1/2
  Linear Terms/1 -> Mux/1
  Linear Reconstruct/1 -> Linear Terms/1, P3/1
  P3/1 -> Mux1/1
  Mux/1 -> recombine/1
  recombine/1 -> Param Rec/1
  Ground/1 -> h/1

== system models2/Reconstruct/logRecon ==
  Param : Inport
  Ground : Ground
  Linear Reconstruct : Gain  Gain=invDG  Multiplication=Matrix(K*u)  SaturateOnIntegerOverflow=on
  Linear Terms : Selector  Elements=LinTerms  InputPortWidth=NTerms
  Mux : Mux  Inputs=2
  Mux1 : Mux  Inputs=2
  Nonlinear  reconstruct : Subsystem
  Nonlinear Terms : Selector  Elements=NLTerm  InputPortWidth=NTerms
  Pn : Selector  Orientation=down  Elements=KnownParam  InputPortWidth=NTerms
  Recombine : Selector  Elements=recombine  InputPortWidth=NTerms
  Param Rec : Outport
  h : Outport  Port=2
  wires:
  Linear Terms/1 -> Mux/1
  Nonlinear  reconstruct/1(k) -> Mux/2
  Param/1 -> Linear Reconstruct/1, Nonlinear Terms/1
  Mux1/1 -> Nonlinear  reconstruct/1(P)
  Nonlinear Terms/1 -> Mux1/2
  Linear Reconstruct/1 -> Linear Terms/1, Pn/1
  Pn/1 -> Mux1/1  "P"
  Mux/1 -> Recombine/1
  Recombine/1 -> Param Rec/1
  Ground/1 -> h/1

== system models2/Reconstruct/mmfRecon ==
  Param : Inport
  Ground : Ground
  Linear Reconstruct : Gain  Gain=invDG  Multiplication=Matrix(K*u)  SaturateOnIntegerOverflow=on
  Linear Terms : Selector  Elements=LinTerms  InputPortWidth=NTerms
  Mux : Mux  Inputs=2
  Nonlinear  reconstruct : Subsystem
  Nonlinear Terms : Selector  Elements=NLTerm  InputPortWidth=NTerms
  Recombine : Selector  Elements=recombine  InputPortWidth=NTerms
  Param Rec : Outport
  h : Outport  Port=2
  wires:
  Param/1 -> Nonlinear Terms/1, Linear Reconstruct/1
  Nonlinear  reconstruct/1(d) -> Mux/2
  Linear Terms/1 -> Mux/1
  Nonlinear Terms/1 -> Nonlinear  reconstruct/1(P)
  Mux/1 -> Recombine/1
  Recombine/1 -> Param Rec/1
  Linear Reconstruct/1 -> Linear Terms/1
  Ground/1 -> h/1

== system models2/Reconstruct/richReconDelta ==
  note: P3
  Param : Inport
  Ground : Ground
  Linear  Reconstruction : Gain  Gain=invDG  Multiplication=Matrix(K*u)  SaturateOnIntegerOverflow=on
  Linear Terms : Selector  Elements=LinTerms  InputPortWidth=NTerms
  Mux : Mux  Inputs=2
  Mux1 : Mux  Inputs=2
  Nonlinear  reconstruct : Subsystem
  Nonlinear Terms : Selector  Elements=NLTerm  InputPortWidth=NTerms
  P3 : Selector  Orientation=down  Elements=[3]  InputPortWidth=NTerms
  Recombine : Selector  Elements=recombine  InputPortWidth=NTerms
  Param Rec : Outport
  h : Outport  Port=2
  wires:
  Linear Terms/1 -> Mux/1
  Nonlinear  reconstruct/1(d) -> Mux/2
  Param/1 -> Linear  Reconstruction/1, Nonlinear Terms/1
  Linear  Reconstruction/1 -> Linear Terms/1, P3/1
  Nonlinear Terms/1 -> Mux1/2
  P3/1 -> Mux1/1
  Mux1/1 -> Nonlinear  reconstruct/1(P)
  Mux/1 -> Recombine/1
  Recombine/1 -> Param Rec/1
  Ground/1 -> h/1

== system models2/Reconstruct/richReconKappa ==
  note: P4
  Param : Inport
  Ground : Ground
  Linear  Reconstruction : Gain  Gain=invDG  Multiplication=Matrix(K*u)  SaturateOnIntegerOverflow=on
  Linear Terms : Selector  Elements=LinTerms  InputPortWidth=NTerms
  Mux : Mux  Inputs=2
  Mux1 : Mux  Inputs=2
  Nonlinear  reconstruct : Subsystem
  Nonlinear Terms : Selector  Elements=NLTerm  InputPortWidth=NTerms
  P4 : Selector  Orientation=down  Elements=[4]  InputPortWidth=NTerms
  Recombine : Selector  Elements=recombine  InputPortWidth=NTerms
  Param Rec : Outport
  h : Outport  Port=2
  wires:
  Ground/1 -> h/1
  Recombine/1 -> Param Rec/1
  Mux/1 -> Recombine/1
  Mux1/1 -> Nonlinear  reconstruct/1(P)
  P4/1 -> Mux1/1
  Nonlinear Terms/1 -> Mux1/2
  Linear  Reconstruction/1 -> P4/1, Linear Terms/1
  Param/1 -> Nonlinear Terms/1, Linear  Reconstruction/1
  Nonlinear  reconstruct/1(d) -> Mux/2
  Linear Terms/1 -> Mux/1

== system models2/Reconstruct/userLocalRecon ==
  Param : Inport
  Ground : Ground
  Linear  Reconstruct : Gain  Gain=invDG  Multiplication=Matrix(K*u)  SaturateOnIntegerOverflow=on
  Nonlinear  reconstruct : Subsystem
  Param Rec : Outport
  h : Outport  Port=2
  wires:
  Ground/1 -> h/1
  Nonlinear  reconstruct/1(p) -> Param Rec/1
  Linear  Reconstruct/1 -> Nonlinear  reconstruct/1(linP)
  Param/1 -> Linear  Reconstruct/1, Nonlinear  reconstruct/2(rf)

== system models2/Reconstruct/weibRecon ==
  note: P4
  Param : Inport
  Ground : Ground
  Linear  Reconstruct : Gain  Gain=invDG  Multiplication=Matrix(K*u)  SaturateOnIntegerOverflow=on
  Linear Terms : Selector  Elements=LinTerms  InputPortWidth=NTerms
  Mux : Mux  Inputs=2
  Mux1 : Mux  Inputs=2
  Nonlinear  reconstruct : Subsystem
  Nonlinear Terms : Selector  Elements=NLTerm  InputPortWidth=NTerms
  P4 : Selector  Orientation=down  Elements=4  InputPortWidth=NTerms
  Recombine : Selector  Elements=recombine  InputPortWidth=NTerms
  Param Rec : Outport
  h : Outport  Port=2
  wires:
  Linear Terms/1 -> Mux/1
  Nonlinear  reconstruct/1(d1) -> Mux/2
  Param/1 -> Linear  Reconstruct/1, Nonlinear Terms/1
  Nonlinear Terms/1 -> Mux1/2
  Mux1/1 -> Nonlinear  reconstruct/1(P1)
  P4/1 -> Mux1/1
  Linear  Reconstruct/1 -> Linear Terms/1, P4/1
  Mux/1 -> Recombine/1
  Recombine/1 -> Param Rec/1
  Ground/1 -> h/1

== system models2/TwoStage/lolimotGaussianEval ==
  X : Inport
  Gain : Gain  Gain=P  Multiplication=Matrix(u*K)  SaturateOnIntegerOverflow=on
  Gaussian : models2/TwoStage/rbfUtils/Gaussian
  Math Function : Math  Operator=transpose  SaturateOnIntegerOverflow=on
  Product : Product  Multiplication=Matrix(*)  SaturateOnIntegerOverflow=on  InputSameDT=on
  Product4 : Product  Multiplication=Matrix(*)  SaturateOnIntegerOverflow=on  InputSameDT=on
  R1 : models2/TwoStage/rbfUtils/R1
  Reshape2 : simulink/Math Operations/Reshape  OutputDimensionality=Column vector  OutputDimensions=[1,1]
  Reshape3 : simulink/Math Operations/Reshape  OutputDimensionality=Row vector  OutputDimensions=[1,1]
  betaModel_x2fx : models2/TwoStage/rbfUtils/betaModel_x2fx
  normaliser : models2/TwoStage/rbfUtils/normaliser
  Y : Outport
  J : Outport  Port=2
  wires:
  Product/1 -> J/1
  Reshape2/1 -> Product/1
  Math Function/1 -> Product4/2  "betas"
  Reshape3/1 -> Gain/1
  X/1 -> R1/1, betaModel_x2fx/1
  R1/1 -> Gaussian/1
  Gaussian/1 -> normaliser/1
  Product4/1 -> Y/1
  betaModel_x2fx/1 -> Reshape2/1, Reshape3/1  "x2fx"
  Gain/1 -> Math Function/1
  normaliser/1 -> Product/2, Product4/1

== system models2/TwoStage/lolimotMultiquadricEval ==
  X : Inport
  Gain : Gain  Gain=P  Multiplication=Matrix(u*K)  SaturateOnIntegerOverflow=on
  Math Function : Math  Operator=transpose  SaturateOnIntegerOverflow=on
  Multiquadric : models2/TwoStage/rbfUtils/Multiquadric
  Product : Product  Multiplication=Matrix(*)  SaturateOnIntegerOverflow=on  InputSameDT=on
  Product4 : Product  Multiplication=Matrix(*)  SaturateOnIntegerOverflow=on  InputSameDT=on
  R1 : models2/TwoStage/rbfUtils/R1
  Reshape2 : simulink/Math Operations/Reshape  OutputDimensionality=Column vector  OutputDimensions=[1,1]
  Reshape3 : simulink/Math Operations/Reshape  OutputDimensionality=Row vector  OutputDimensions=[1,1]
  betaModel_x2fx : models2/TwoStage/rbfUtils/betaModel_x2fx
  normaliser : models2/TwoStage/rbfUtils/normaliser
  Y : Outport
  J : Outport  Port=2
  wires:
  normaliser/1 -> Product4/1, Product/2
  Gain/1 -> Math Function/1
  betaModel_x2fx/1 -> Reshape3/1, Reshape2/1  "x2fx"
  Product4/1 -> Y/1
  Multiquadric/1 -> normaliser/1
  R1/1 -> Multiquadric/1
  X/1 -> R1/1, betaModel_x2fx/1
  Reshape3/1 -> Gain/1
  Math Function/1 -> Product4/2  "betas"
  Reshape2/1 -> Product/1
  Product/1 -> J/1

== system models2/TwoStage/lolimotRecmultiquadricEval ==
  X : Inport
  Gain : Gain  Gain=P  Multiplication=Matrix(u*K)  SaturateOnIntegerOverflow=on
  Math Function : Math  Operator=transpose  SaturateOnIntegerOverflow=on
  Product : Product  Multiplication=Matrix(*)  SaturateOnIntegerOverflow=on  InputSameDT=on
  Product4 : Product  Multiplication=Matrix(*)  SaturateOnIntegerOverflow=on  InputSameDT=on
  R1 : models2/TwoStage/rbfUtils/R1
  RecMultiquadric : models2/TwoStage/rbfUtils/RecMultiquadric
  Reshape2 : simulink/Math Operations/Reshape  OutputDimensionality=Column vector  OutputDimensions=[1,1]
  Reshape3 : simulink/Math Operations/Reshape  OutputDimensionality=Row vector  OutputDimensions=[1,1]
  betaModel_x2fx : models2/TwoStage/rbfUtils/betaModel_x2fx
  normaliser : models2/TwoStage/rbfUtils/normaliser
  Y : Outport
  J : Outport  Port=2
  wires:
  Product/1 -> J/1
  Reshape2/1 -> Product/1
  Math Function/1 -> Product4/2  "betas"
  Reshape3/1 -> Gain/1
  X/1 -> R1/1, betaModel_x2fx/1
  R1/1 -> RecMultiquadric/1
  RecMultiquadric/1 -> normaliser/1
  Product4/1 -> Y/1
  betaModel_x2fx/1 -> Reshape2/1, Reshape3/1  "x2fx"
  Gain/1 -> Math Function/1
  normaliser/1 -> Product/2, Product4/1

== system models2/TwoStage/lolimotWendlandEval ==
  X : Inport
  Constant : Constant  Value=WP
  Constant1 : Constant  Value=E
  Gain : Gain  Gain=P  Multiplication=Matrix(u*K)  SaturateOnIntegerOverflow=on
  Math Function : Math  Operator=transpose  SaturateOnIntegerOverflow=on
  Math Function1 : Math  Operator=sqrt  SaturateOnIntegerOverflow=on
  Product : Product  Multiplication=Matrix(*)  SaturateOnIntegerOverflow=on  InputSameDT=on
  Product4 : Product  Multiplication=Matrix(*)  SaturateOnIntegerOverflow=on  InputSameDT=on
  R1 : models2/TwoStage/rbfUtils/R1
  Reshape2 : simulink/Math Operations/Reshape  OutputDimensionality=Column vector  OutputDimensions=[1,1]
  Reshape3 : simulink/Math Operations/Reshape  OutputDimensionality=Row vector  OutputDimensions=[1,1]
  Wendland : models2/TwoStage/rbfUtils/Wendland  NumTerms=WendlandNumTerms
  betaModel_x2fx : models2/TwoStage/rbfUtils/betaModel_x2fx
  normaliser : models2/TwoStage/rbfUtils/normaliser
  Y : Outport
  J : Outport  Port=2
  wires:
  Math Function1/1 -> Wendland/1
  R1/1 -> Math Function1/1
  Constant1/1 -> Wendland/3
  Constant/1 -> Wendland/2
  normaliser/1 -> Product4/1, Product/2
  Gain/1 -> Math Function/1
  betaModel_x2fx/1 -> Reshape3/1, Reshape2/1  "x2fx"
  Product4/1 -> Y/1
  Wendland/1 -> normaliser/1
  X/1 -> R1/1, betaModel_x2fx/1
  Reshape3/1 -> Gain/1
  Math Function/1 -> Product4/2  "betas"
  Reshape2/1 -> Product/1
  Product/1 -> J/1

== system models2/TwoStage/mvCubicEval ==
  X : Inport
  Constant : Constant  Value=coeffs
  S-Function : S-Function  FunctionName=mvCubicEvalSFnV2  Parameters=orderM, reorderM, interact  SFunctionModules=mvcubiceval_helper
  Y : Outport
  wires:
  Constant/1 -> S-Function/1
  S-Function/1 -> Y/1
  X/1 -> S-Function/2

== system models2/TwoStage/rbfCubicEval ==
  X : Inport
  Constant1 : Constant  Value=S  VectorParams1D=off
  Constant2 : Constant  Value=C  VectorParams1D=off
  Constant3 : Constant  Value=B
  Cube : Product  Inputs=3  SaturateOnIntegerOverflow=on
  Math Function : Math  Operator=sqrt  SaturateOnIntegerOverflow=on
  Product4 : Product  Multiplication=Matrix(*)  SaturateOnIntegerOverflow=on  InputSameDT=on
  R : models2/TwoStage/rbfUtils/R
  Y : Outport
  J : Outport  Port=2
  wires:
  Constant3/1 -> Product4/2
  Product4/1 -> Y/1
  Constant2/1 -> R/2
  X/1 -> R/1
  Constant1/1 -> R/3
  R/1 -> Math Function/1
  Math Function/1 -> Cube/2, Cube/1, Cube/3
  Cube/1 -> Product4/1, J/1

== system models2/TwoStage/rbfGaussianEval ==
  X : Inport
  Constant1 : Constant  Value=S  VectorParams1D=off
  Constant2 : Constant  Value=C  VectorParams1D=off
  Constant3 : Constant  Value=B
  Gaussian : models2/TwoStage/rbfUtils/Gaussian
  Product4 : Product  Multiplication=Matrix(*)  SaturateOnIntegerOverflow=on  InputSameDT=on
  R : models2/TwoStage/rbfUtils/R
  Y : Outport
  J : Outport  Port=2
  wires:
  Product4/1 -> Y/1
  Constant2/1 -> R/2
  Gaussian/1 -> J/1, Product4/1
  R/1 -> Gaussian/1
  X/1 -> R/1
  Constant3/1 -> Product4/2
  Constant1/1 -> R/3

== system models2/TwoStage/rbfLinearEval ==
  X : Inport
  Constant1 : Constant  Value=S  VectorParams1D=off
  Constant2 : Constant  Value=C  VectorParams1D=off
  Constant3 : Constant  Value=B
  Math Function : Math  Operator=sqrt  SaturateOnIntegerOverflow=on
  Product4 : Product  Multiplication=Matrix(*)  SaturateOnIntegerOverflow=on  InputSameDT=on
  R : models2/TwoStage/rbfUtils/R
  Y : Outport
  J : Outport  Port=2
  wires:
  R/1 -> Math Function/1
  Constant1/1 -> R/3
  X/1 -> R/1
  Constant2/1 -> R/2
  Product4/1 -> Y/1
  Math Function/1 -> Product4/1, J/1
  Constant3/1 -> Product4/2
